simulink model "Manipulator_PDControl"  (R2020b)
settings: Solver=FixedStepAuto  StartTime=0.0  StopTime=t_final  FixedStep=dt  RelTol=1e-3
values from neighbouring files (symbols this model uses):
  dq_0 = 0.1 *[ 0  -1  0]    [Initialization.m]
  q_0 = [0;-0.9;2.7]    [Initialization.m]
settings Model: Creator=m2aali  LastModifiedBy=Kons

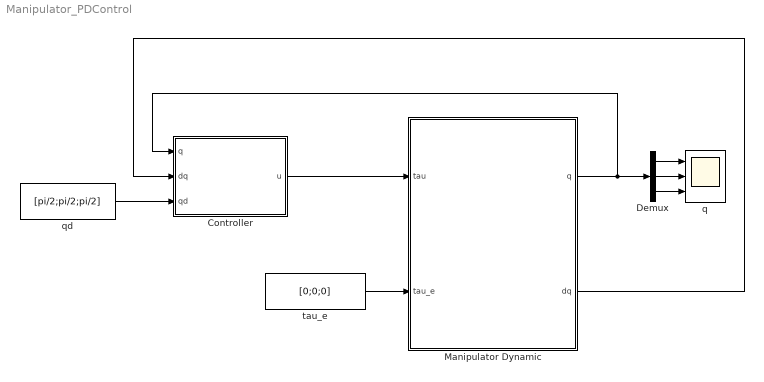
== system Manipulator_PDControl ==
  Controller : Subsystem
  Demux : Demux  Outputs=3
  Manipulator Dynamic : Subsystem
  q : Scope  NumInputPorts=3
  qd : Constant  Value=[pi/2;pi/2;pi/2]
  tau_e : Constant  Value=[0;0;0]
  wires:
  tau_e/1 -> Manipulator Dynamic/2(tau_e)
  Manipulator Dynamic/1(q) -> Demux/1, Controller/1(q)
  qd/1 -> Controller/3(qd)
  Manipulator Dynamic/2(dq) -> Controller/2(dq)
  Controller/1(u) -> Manipulator Dynamic/1(tau)
  Demux/1 -> q/1
  Demux/2 -> q/2
  Demux/3 -> q/3

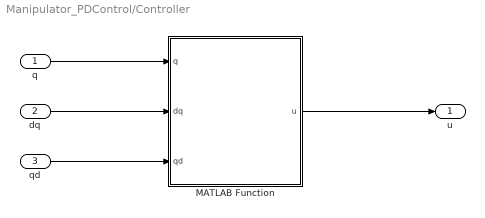
== system Manipulator_PDControl/Controller ==
  q : Inport
  dq : Inport  Port=2
  qd : Inport  Port=3
  MATLAB Function : MATLAB Function  TreatAsAtomicUnit=on
  u : Outport
  wires:
  dq/1 -> MATLAB Function/2(dq)
  MATLAB Function/1(u) -> u/1
  qd/1 -> MATLAB Function/3(qd)
  q/1 -> MATLAB Function/1(q)

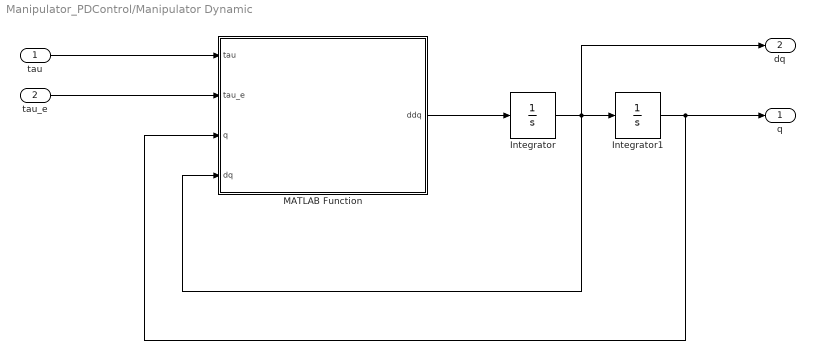
== system Manipulator_PDControl/Manipulator Dynamic ==
  tau : Inport
  tau_e : Inport  Port=2
  Integrator : Integrator  InitialCondition=dq_0
  Integrator1 : Integrator  InitialCondition=q_0
  MATLAB Function : MATLAB Function  TreatAsAtomicUnit=on
  q : Outport
  dq : Outport  Port=2
  wires:
  MATLAB Function/1(ddq) -> Integrator/1
  tau/1 -> MATLAB Function/1(tau)
  tau_e/1 -> MATLAB Function/2(tau_e)
  Integrator1/1 -> q/1, MATLAB Function/3(q)
  Integrator/1 -> dq/1, MATLAB Function/4(dq), Integrator1/1

== matlab function Manipulator_PDControl/Controller/MATLAB Function ==
  data: q input; dq input; u output; qd input
function u = fcn(q, dq, qd)
% PD + gravity compensation controller function

%% general physical parameters

l1 = 0.6731;
l2 = 0.432;
l3 = 0.434;
lc2 = 0.216;
lc3 = 0.164;
m2 = 15.46;
m3 = 9.55;
J = 0.302;

%% Joint Space variables

q1 = q(1);
q2 = q(2);
q3 = q(3);

dq1 = dq(1);
dq2 = dq(2);
dq3 = dq(3);
g = 9.81;

%% Vector of Potential Forces Parameters

g21 = -g * (lc3 * m3 * sin(q2 + q3) + lc2 * m2 * cos(q2) + l2 * m3 * cos(q2));
g31 = -g * (lc3 * m3 * sin(q2 + q3));

G = [0;
    g21;
    g31];

%% PD Controller Parameters 

Kp = [20,0,0; 0, 10 ,0; 0, 0 , 10];  %  Kp is 3*3 matrix of proportional gain 
Kd = [1,0,0; 0, 1 ,0; 0, 0 , 1]; %Kd is 3*3 matrix of derivative gain

%% Control law

u = - Kp * (q - qd) - Kd * dq + G;

== matlab function Manipulator_PDControl/Manipulator Dynamic/MATLAB Function ==
  data: tau input; tau_e input; q input; ddq output; dq input
function ddq = DynamicModel( tau, tau_e, q, dq)
%%%%%
% 3-DOF Puma-560 Dynamic Model Function
% H(q)* ddq + C(q) * dq + G = tau + tau_e
% q is 3*1 vector of joint variables (radian)
% H(q) is the inertia matrix
% C(q) is the matrix of Coriolis and centrifugal forces
% G(q) is  the vector of potential forces Parameters
% tau is control torque 
% tau_e is the external torque due to the interaction with the environment
%%%%%

%% Joint Space variables

q1 = q(1);
q2 = q(2);
q3 = q(3);

dq1 = dq(1);
dq2 = dq(2);
dq3 = dq(3);

%% general physical parameters

l1 = 0.6731;
l2 = 0.432;
l3 = 0.434;
lc2 = 0.216;
lc3 = 0.164;
m2 = 15.46;
m3 = 9.55;
J = 0.302;

%% Inertia Matrix Parameters

J1 = m3 * lc3^2;
J12 = (m2 * lc2^2) + (m3 * l2^2);
J13 = l2 * lc3 * m3;


h11 = J + J1 * (sin(q2 + q3))^2 + J12 * (cos(q2))^2 + 2 * J13 * cos(q2) * sin(q2+q3);
h22 = J1 + J12 + 2 * J13 * sin(q3);
h23 = J1 + J13 * sin(q3);
h32 = h23;
h33 = J1;

H = [h11, 0 ,0 ;
    0 , h22, h23;
    0 , h32, h33];

%% Coriolis Matrix Parameters

c12_1 = J1 * sin(2 * (q1 + q2)) - J12 * sin(2 * q2) + 2 * J13 * cos(2 * q2 +q3);
c13_1 = J1 * sin(2 * (q2 + q3)) + 2 * J13 * cos(q2) * cos(q2 + q3);
c11_2 = (1/2) * (-J1 * sin(2 * (q2 + q3)) + J12 * sin(2 * q2) - 2 * J13 * cos(2 * q2 + q3));
c22_2 = 2 * J13 * cos(q3);
c23_2 = J13 * cos(q3);
c22_3 = -J13 * cos(q3) * dq2;
c11_3 = (-1/2) * (J1 * sin(2 * (q2 + q3)) + J13 * cos(q2) * cos(q2 + q3));

C = [0, c12_1 * dq1, c13_1 * dq3;
    c11_2 * dq1, 0 , c22_2 * dq2 + c23_2 * dq3;
    c11_3 * dq1, c22_3 * dq2, 0];

%% Vector of Potential Forces Parameters

g = 9.81;

g21 = -g * (lc3 * m3 * sin(q2 + q3) + lc2 * m2 * cos(q2) + l2 * m3 * cos(q2));
g31 = -g * (lc3 * m3 * sin(q2 + q3));

G = [0;
    g21;
    g31];

%% Function output

ddq = inv(H)*(tau + tau_e - C * dq - G);
